simulink model "GPC_conROS_Comparacion"  (R2023a)
settings: Solver=FixedStepAuto  StartTime=0.0  StopTime=50  FixedStep=0.01  RelTol=1e-3
settings Model: Creator=carlo  LastModifiedBy=camarin
settings OptimizationCC: EnhancedBackFolding=on  PassReuseOutputArgsThreshold=0  MaxStackSize=64  OptimizeBlockOrder=speed  DifferentSizesBufferReuse=on
settings DebuggingCC: ParameterTunabilityLossMsg=error  UnconnectedInputMsg=warning  UnconnectedOutputMsg=warning  UnconnectedLineMsg=warning
settings HardwareCC: ProdBitPerLong=64  ProdHWDeviceType=Intel->x86-64 (Linux 64)  UseEmbeddedCoderFeatures=off
settings ModelReferenceCC: EnableRefExpFcnMdlSchedulingChecks=on
settings SFSimCC: MATLABDynamicMemAlloc=off
settings RTWCC: Description=Embedded Coder  SystemTargetFile=ert.tlc  HardwareBoard=Robot Operating System (ROS)  TLCOptions="-aInlineSetEventsForThisBaseRateFcn=TLC_FALSE -aSuppressMultiTaskScheduler=TLC_FALSE  -aRateBasedStepFcn=0"  TemplateMakefile=ert_default_tmf  Toolchain=Catkin  TargetLang=C++  DLArmComputeVersion=19.05
settings CodeAppCC: ForceParamTrailComments=on  OperatorAnnotations=on
settings ERTTargetCC: ERTCustomFileBanners=off  SupportContinuousTime=on  SupportNonInlinedSFcns=on  RemoveResetFunc=off  ModelStepFunctionPrototypeControlCompliant=off

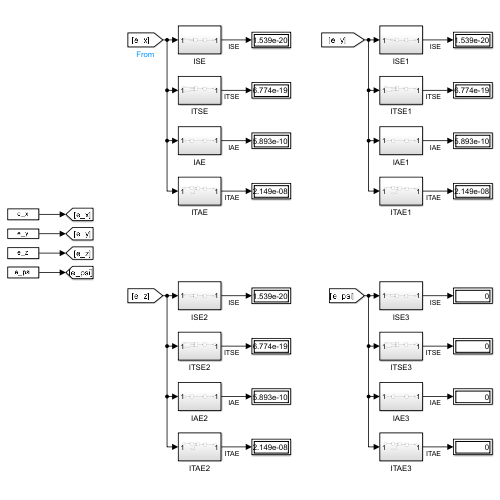
[thumbnail: Simulink's stored preview of the top-level diagram]
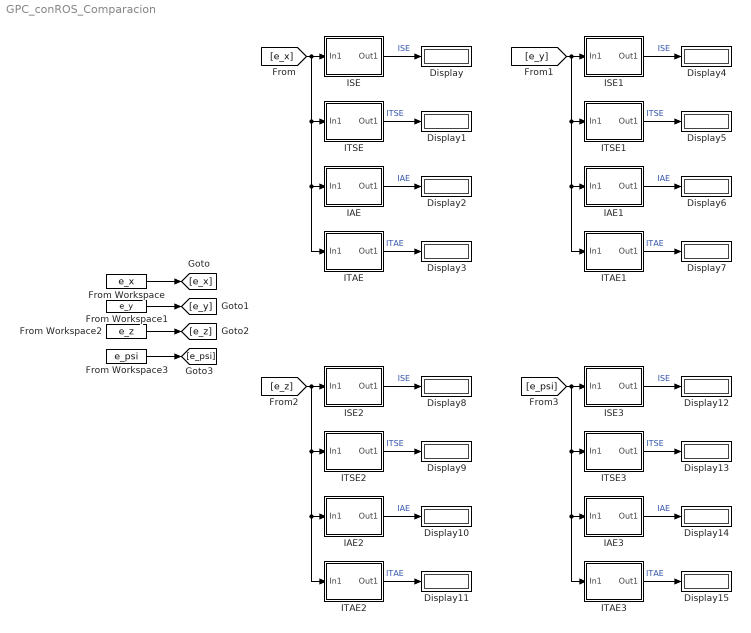
== system GPC_conROS_Comparacion ==
  Display{,1..15} (16 alike) : Display
  From Workspace : FromWorkspace  VariableName=e_x  SampleTime=-1
  From Workspace1 : FromWorkspace  VariableName=e_y  SampleTime=-1
  From Workspace2 : FromWorkspace  VariableName=e_z  SampleTime=-1
  From Workspace3 : FromWorkspace  VariableName=e_psi  SampleTime=-1
  IAE : Subsystem
  IAE1 : Subsystem
  IAE2 : Subsystem
  IAE3 : Subsystem
  ISE : Subsystem
  ISE1 : Subsystem
  ISE2 : Subsystem
  ISE3 : Subsystem
  ITAE : Subsystem
  ITAE1 : Subsystem
  ITAE2 : Subsystem
  ITAE3 : Subsystem
  ITSE : Subsystem
  ITSE1 : Subsystem
  ITSE2 : Subsystem
  ITSE3 : Subsystem
  wires:
  From Workspace/1 -> [e_x]
  ISE1/1(Out1) -> Display4/1  "ISE"
  ITSE/1(Out1) -> Display1/1  "ITSE"
  [e_psi] -> ITAE3/1(In1), IAE3/1(In1), ITSE3/1(In1), ISE3/1(In1)
  ITAE3/1(Out1) -> Display15/1  "ITAE"
  ISE2/1(Out1) -> Display8/1  "ISE"
  [e_y] -> ITAE1/1(In1), IAE1/1(In1), ITSE1/1(In1), ISE1/1(In1)
  ISE3/1(Out1) -> Display12/1  "ISE"
  ISE/1(Out1) -> Display/1  "ISE"
  ITAE/1(Out1) -> Display3/1  "ITAE"
  ITSE1/1(Out1) -> Display5/1  "ITSE"
  [e_x] -> ITAE/1(In1), IAE/1(In1), ITSE/1(In1), ISE/1(In1)
  ITAE2/1(Out1) -> Display11/1  "ITAE"
  IAE/1(Out1) -> Display2/1  "IAE"
  IAE3/1(Out1) -> Display14/1  "IAE"
  ITSE2/1(Out1) -> Display9/1  "ITSE"
  IAE1/1(Out1) -> Display6/1  "IAE"
  ITAE1/1(Out1) -> Display7/1  "ITAE"
  ITSE3/1(Out1) -> Display13/1  "ITSE"
  IAE2/1(Out1) -> Display10/1  "IAE"
  [e_z] -> ITAE2/1(In1), IAE2/1(In1), ITSE2/1(In1), ISE2/1(In1)
  From Workspace2/1 -> [e_z]
  From Workspace1/1 -> [e_y]
  From Workspace3/1 -> [e_psi]

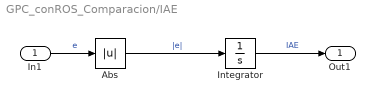
== system GPC_conROS_Comparacion/IAE ==
  In1 : Inport
  Abs : Abs  SaturateOnIntegerOverflow=off
  Integrator : Integrator
  Out1 : Outport
  wires:
  Integrator/1 -> Out1/1  "IAE"
  In1/1 -> Abs/1  "e"
  Abs/1 -> Integrator/1  "|e|"

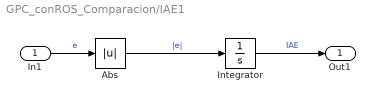
== system GPC_conROS_Comparacion/IAE1 ==
  In1 : Inport
  Abs : Abs  SaturateOnIntegerOverflow=off
  Integrator : Integrator
  Out1 : Outport
  wires:
  Integrator/1 -> Out1/1  "IAE"
  In1/1 -> Abs/1  "e"
  Abs/1 -> Integrator/1  "|e|"

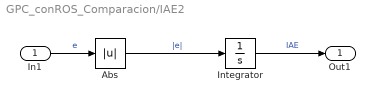
== system GPC_conROS_Comparacion/IAE2 ==
  In1 : Inport
  Abs : Abs  SaturateOnIntegerOverflow=off
  Integrator : Integrator
  Out1 : Outport
  wires:
  Integrator/1 -> Out1/1  "IAE"
  In1/1 -> Abs/1  "e"
  Abs/1 -> Integrator/1  "|e|"

== system GPC_conROS_Comparacion/IAE3 ==
  In1 : Inport
  Abs : Abs  SaturateOnIntegerOverflow=off
  Integrator : Integrator
  Out1 : Outport
  wires:
  Integrator/1 -> Out1/1  "IAE"
  In1/1 -> Abs/1  "e"
  Abs/1 -> Integrator/1  "|e|"

== system GPC_conROS_Comparacion/ISE ==
  In1 : Inport
  Integrator : Integrator
  Product : Product
  Out1 : Outport
  wires:
  In1/1 -> Product/2, Product/1  "e"
  Product/1 -> Integrator/1  "e^2"
  Integrator/1 -> Out1/1  "ISE"

== system GPC_conROS_Comparacion/ISE1 ==
  In1 : Inport
  Integrator : Integrator
  Product : Product
  Out1 : Outport
  wires:
  In1/1 -> Product/2, Product/1  "e"
  Product/1 -> Integrator/1  "e^2"
  Integrator/1 -> Out1/1  "ISE"

== system GPC_conROS_Comparacion/ISE2 ==
  In1 : Inport
  Integrator : Integrator
  Product : Product
  Out1 : Outport
  wires:
  In1/1 -> Product/2, Product/1  "e"
  Product/1 -> Integrator/1  "e^2"
  Integrator/1 -> Out1/1  "ISE"

== system GPC_conROS_Comparacion/ISE3 ==
  In1 : Inport
  Integrator : Integrator
  Product : Product
  Out1 : Outport
  wires:
  In1/1 -> Product/2, Product/1  "e"
  Product/1 -> Integrator/1  "e^2"
  Integrator/1 -> Out1/1  "ISE"

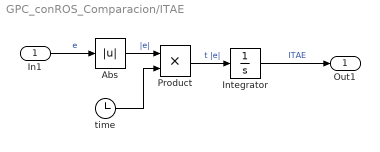
== system GPC_conROS_Comparacion/ITAE ==
  In1 : Inport
  Abs : Abs  SaturateOnIntegerOverflow=off
  Integrator : Integrator
  Product : Product
  time : Clock
  Out1 : Outport
  wires:
  In1/1 -> Abs/1  "e"
  Integrator/1 -> Out1/1  "ITAE"
  time/1 -> Product/2
  Abs/1 -> Product/1  "|e|"
  Product/1 -> Integrator/1  "t |e|"

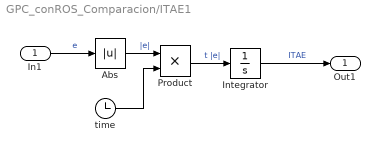
== system GPC_conROS_Comparacion/ITAE1 ==
  In1 : Inport
  Abs : Abs  SaturateOnIntegerOverflow=off
  Integrator : Integrator
  Product : Product
  time : Clock
  Out1 : Outport
  wires:
  In1/1 -> Abs/1  "e"
  Integrator/1 -> Out1/1  "ITAE"
  time/1 -> Product/2
  Abs/1 -> Product/1  "|e|"
  Product/1 -> Integrator/1  "t |e|"

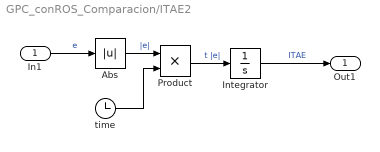
== system GPC_conROS_Comparacion/ITAE2 ==
  In1 : Inport
  Abs : Abs  SaturateOnIntegerOverflow=off
  Integrator : Integrator
  Product : Product
  time : Clock
  Out1 : Outport
  wires:
  In1/1 -> Abs/1  "e"
  Integrator/1 -> Out1/1  "ITAE"
  time/1 -> Product/2
  Abs/1 -> Product/1  "|e|"
  Product/1 -> Integrator/1  "t |e|"

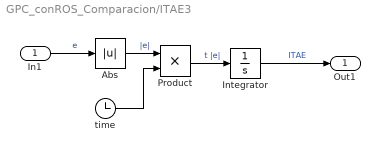
== system GPC_conROS_Comparacion/ITAE3 ==
  In1 : Inport
  Abs : Abs  SaturateOnIntegerOverflow=off
  Integrator : Integrator
  Product : Product
  time : Clock
  Out1 : Outport
  wires:
  In1/1 -> Abs/1  "e"
  Integrator/1 -> Out1/1  "ITAE"
  time/1 -> Product/2
  Abs/1 -> Product/1  "|e|"
  Product/1 -> Integrator/1  "t |e|"

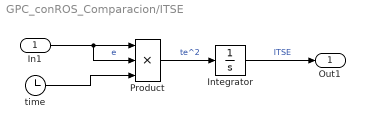
== system GPC_conROS_Comparacion/ITSE ==
  In1 : Inport
  Integrator : Integrator
  Product : Product  Inputs=3
  time : Clock
  Out1 : Outport
  wires:
  Integrator/1 -> Out1/1  "ITSE"
  In1/1 -> Product/1, Product/2  "e"
  time/1 -> Product/3
  Product/1 -> Integrator/1  "te^2"

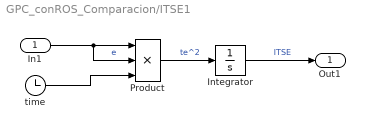
== system GPC_conROS_Comparacion/ITSE1 ==
  In1 : Inport
  Integrator : Integrator
  Product : Product  Inputs=3
  time : Clock
  Out1 : Outport
  wires:
  Integrator/1 -> Out1/1  "ITSE"
  In1/1 -> Product/1, Product/2  "e"
  time/1 -> Product/3
  Product/1 -> Integrator/1  "te^2"

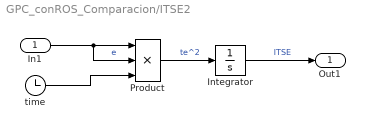
== system GPC_conROS_Comparacion/ITSE2 ==
  In1 : Inport
  Integrator : Integrator
  Product : Product  Inputs=3
  time : Clock
  Out1 : Outport
  wires:
  Integrator/1 -> Out1/1  "ITSE"
  In1/1 -> Product/1, Product/2  "e"
  time/1 -> Product/3
  Product/1 -> Integrator/1  "te^2"

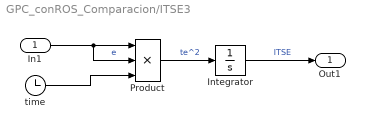
== system GPC_conROS_Comparacion/ITSE3 ==
  In1 : Inport
  Integrator : Integrator
  Product : Product  Inputs=3
  time : Clock
  Out1 : Outport
  wires:
  Integrator/1 -> Out1/1  "ITSE"
  In1/1 -> Product/1, Product/2  "e"
  time/1 -> Product/3
  Product/1 -> Integrator/1  "te^2"
